simulink model "Standard_Control"  (Simulink 7.5)
settings: Solver=ode45  StartTime=0.0  StopTime=10.0  RelTol=1e-3
undefined symbols (not defined in the file): ctrller
settings Model: Creator=sriddle  LastModifiedBy=sriddle
settings OptimizationCC: ExpressionDepthLimit=128
settings CodeAppCC: CustomSymbolStrType=$N$R$M_T
settings GRTTargetCC: CombineOutputUpdateFcns=on

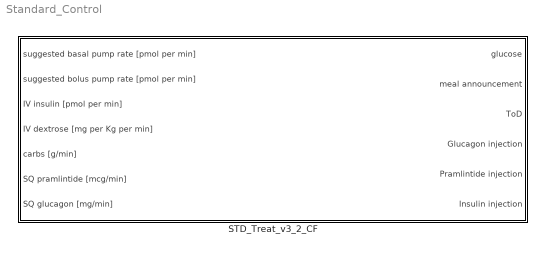
== system Standard_Control ==
  STD_Treat_v3_2_CF : Subsystem

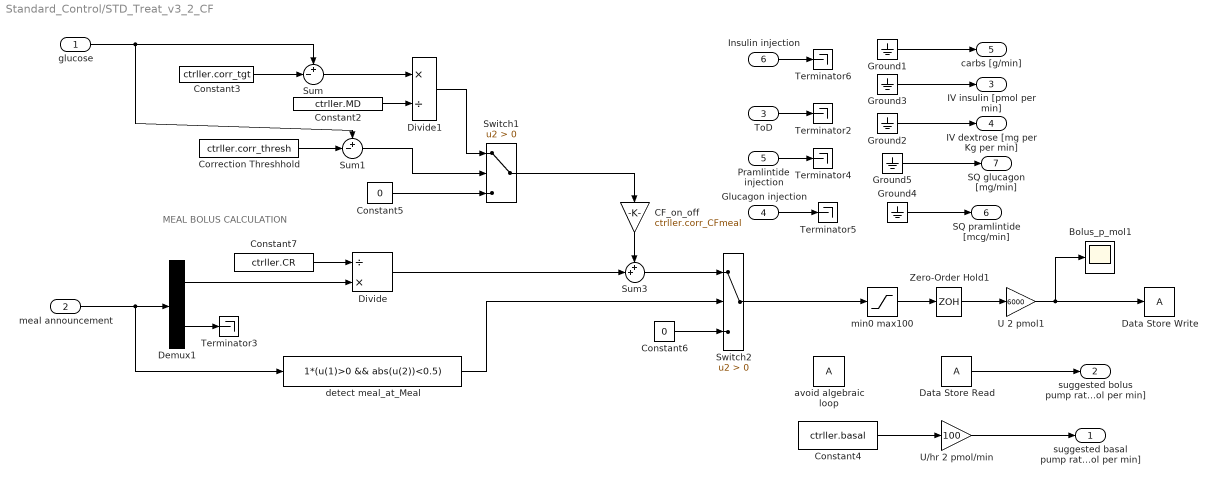
== system Standard_Control/STD_Treat_v3_2_CF ==
  note: MEAL BOLUS CALCULATION
  glucose : Inport
  meal announcement : Inport  Port=2
  ToD : Inport  Port=3
  Glucagon injection : Inport  Port=4
  Pramlintide injection : Inport  Port=5
  Insulin injection : Inport  Port=6
  Bolus_p_mol1 : Scope
      settings: YMin=0  YMax=60000  SaveName=ScopeData5
  CF_on_off : Gain  Gain=ctrller.corr_CFmeal
  Constant2 : Constant  Value=ctrller.MD
  Constant3 : Constant  Value=ctrller.corr_tgt
  Constant4 : Constant  Value=ctrller.basal
  Constant5 : Constant  Value=0
  Constant6 : Constant  Value=0
  Constant7 : Constant  Value=ctrller.CR
  Correction Threshhold : Constant  Value=ctrller.corr_thresh
  Data Store Read : DataStoreRead  DataStoreName=A  SampleTime=0
  Data Store Write : DataStoreWrite  DataStoreName=A  SampleTime=-1
  Demux1 : Demux  Outputs=2
  Divide : Product  Inputs=/*
  Divide1 : Product  Inputs=*/
  Ground{1..5} (5 alike) : Ground
  Sum : Sum  Inputs=+-|
  Sum1 : Sum  Inputs=+-|
  Sum3 : Sum  Inputs=++|
  Switch1 : Switch  Criteria=u2 > Threshold
  Switch2 : Switch  Criteria=u2 > Threshold
  Terminator{2..6} (5 alike) : Terminator
  U 2 pmol1 : Gain  Gain=6000
  U/hr 2 pmol/min : Gain  Gain=100
  Zero-Order Hold1 : ZeroOrderHold
  avoid algebraic loop : DataStoreMemory  DataStoreName=A  ReadBeforeWriteMsg=warning  WriteAfterWriteMsg=warning  WriteAfterReadMsg=warning
  detect meal_at_Meal : Fcn  Expr=1*(u(1)>0 && abs(u(2))<0.5)
  min0 max100 : Saturate  UpperLimit=100  LowerLimit=0
  suggested basal pump rate [pmol per min] : Outport
  suggested bolus pump rate [pmol per min] : Outport  Port=2
  IV insulin [pmol per min] : Outport  Port=3
  IV dextrose [mg per Kg per min] : Outport  Port=4
  carbs [g/min] : Outport  Port=5
  SQ pramlintide [mcg/min] : Outport  Port=6
  SQ glucagon [mg/min] : Outport  Port=7
  wires:
  Data Store Read/1 -> suggested bolus pump rate [pmol per min]/1
  U/hr 2 pmol/min/1 -> suggested basal pump rate [pmol per min]/1
  Constant4/1 -> U/hr 2 pmol/min/1
  ToD/1 -> Terminator2/1
  Constant6/1 -> Switch2/3
  detect meal_at_Meal/1 -> Switch2/2
  Constant7/1 -> Divide/1
  Demux1/1 -> Divide/2
  meal announcement/1 -> Demux1/1, detect meal_at_Meal/1
  Demux1/2 -> Terminator3/1
  Divide/1 -> Sum3/2
  Zero-Order Hold1/1 -> U 2 pmol1/1
  U 2 pmol1/1 -> Data Store Write/1, Bolus_p_mol1/1
  min0 max100/1 -> Zero-Order Hold1/1
  Ground5/1 -> SQ glucagon [mg/min]/1
  Ground4/1 -> SQ pramlintide [mcg/min]/1
  Pramlintide injection/1 -> Terminator4/1
  Ground2/1 -> IV dextrose [mg per Kg per min]/1
  Glucagon injection/1 -> Terminator5/1
  Ground1/1 -> carbs [g/min]/1
  Ground3/1 -> IV insulin [pmol per min]/1
  Insulin injection/1 -> Terminator6/1
  Switch2/1 -> min0 max100/1
  Sum1/1 -> Switch1/2
  Correction Threshhold/1 -> Sum1/2
  Constant5/1 -> Switch1/3
  Switch1/1 -> CF_on_off/1
  Divide1/1 -> Switch1/1
  Constant2/1 -> Divide1/2
  Sum/1 -> Divide1/1
  Constant3/1 -> Sum/2
  glucose/1 -> Sum/1, Sum1/1
  CF_on_off/1 -> Sum3/1
  Sum3/1 -> Switch2/1
